simulink model "UncorSys_Sim"  (R2018b)
settings: Solver=VariableStepAuto  StartTime=0.0  StopTime=10.0  RelTol=1e-3
settings Model: Creator=optiplex3060  LastModifiedBy=optiplex3060

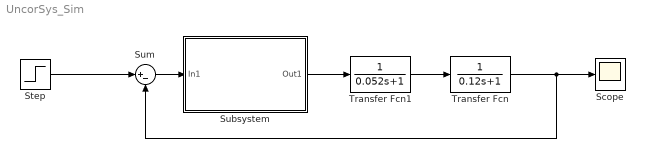
== system UncorSys_Sim ==
  Scope : Scope
  Step : Step  After=2000  SampleTime=0
  Subsystem : Subsystem  mask{Kp=0, Ki=0, Kd=0}
      mask help: PID Controller.
      mask Display: disp('PID')
  Sum : Sum  Inputs=|+-
  Transfer Fcn : TransferFcn  Denominator=[0.12 1]
  Transfer Fcn1 : TransferFcn  Denominator=[0.052 1]
  wires:
  Step/1 -> Sum/1
  Transfer Fcn1/1 -> Transfer Fcn/1
  Transfer Fcn/1 -> Sum/2, Scope/1
  Sum/1 -> Subsystem/1(In1)
  Subsystem/1(Out1) -> Transfer Fcn1/1

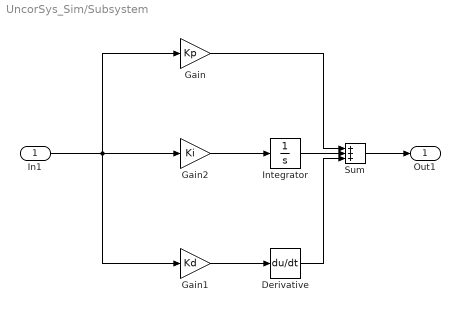
== system UncorSys_Sim/Subsystem ==
  In1 : Inport
  Derivative : Derivative
  Gain : Gain  Gain=Kp
  Gain1 : Gain  Gain=Kd
  Gain2 : Gain  Gain=Ki
  Integrator : Integrator
  Sum : Sum  Inputs=+++
  Out1 : Outport
  wires:
  In1/1 -> Gain1/1, Gain/1, Gain2/1
  Gain2/1 -> Integrator/1
  Integrator/1 -> Sum/2
  Sum/1 -> Out1/1
  Gain/1 -> Sum/1
  Gain1/1 -> Derivative/1
  Derivative/1 -> Sum/3
